simulink model "TPS_Failure_Sys"  (R2020a)
settings: Solver=FixedStepDiscrete  StartTime=0.0  StopTime=10.0  FixedStep=.2  RelTol=1e-3
settings Model: Creator=Administrator  LastModifiedBy=Administrator
settings OptimizationCC: DefaultParameterBehavior=Inlined  EnhancedBackFolding=on  PassReuseOutputArgsAs=Individual arguments  ZeroExternalMemoryAtStartup=off  ZeroInternalMemoryAtStartup=off  OptimizeBlockOrder=speed  DifferentSizesBufferReuse=on  OptimizationCustomize=off  EfficientTunableParamExpr=on
settings DebuggingCC: ParameterTunabilityLossMsg=error
settings HardwareCC: ProdBitPerPointer=32  ProdBitPerSizeT=32  ProdBitPerPtrDiffT=32  ProdLargestAtomicInteger=Long  ProdLargestAtomicFloat=Double  ProdWordSize=32  ProdHWDeviceType=ARM Compatible->ARM Cortex
settings SFSimCC: MATLABDynamicMemAlloc=off
settings RTWCC: SystemTargetFile=ert.tlc  GenCodeOnly=on  TemplateMakefile=ert_default_tmf
settings CodeAppCC: ForceParamTrailComments=on  IgnoreCustomStorageClasses=off  OperatorAnnotations=on  SimulinkDataObjDesc=on  SFDataObjDesc=on  InsertBlockDesc=on
settings ERTTargetCC: TargetLangStandard=C99 (ISO)  GenerateSampleERTMain=on  InlinedParameterPlacement=NonHierarchical  ERTCustomFileTemplate=example_file_process.tlc

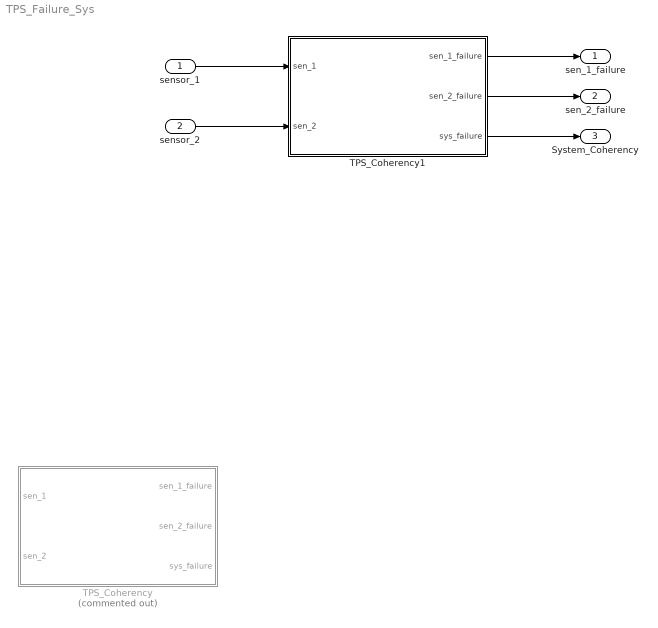
== system TPS_Failure_Sys ==
  sensor_1 : Inport
  sensor_2 : Inport  Port=2
  TPS_Coherency : Stateflow chart  Commented=on  TreatAsAtomicUnit=on
  TPS_Coherency1 : Stateflow chart  TreatAsAtomicUnit=on
  sen_1_failure : Outport
  sen_2_failure : Outport  Port=2
  System_Coherency : Outport  Port=3
  wires:
  sensor_2/1 -> TPS_Coherency1/2(sen_2)
  sensor_1/1 -> TPS_Coherency1/1(sen_1)
  TPS_Coherency1/2(sen_2_failure) -> sen_2_failure/1
  TPS_Coherency1/3(sys_failure) -> System_Coherency/1
  TPS_Coherency1/1(sen_1_failure) -> sen_1_failure/1

== stateflow chart TPS_Failure_Sys/TPS_Coherency1 ==
  state sen2 [parallel]
    settings: executionOrder=3
    (default) -> (junction 112)
    (junction 112) -> (junction 111) [order 1] : [sen_2<.5 || sen_2>4.5]
    sen2 -> (junction 112)
    (junction 111) -> (junction 102) : {sen_2_failure=1}
    (junction 112) -> (junction 105) [order 2] : {sen_2_failure=0}
    (junction 105) -> (junction 102)
    (junction 102) -> (junction 110)
  state sen1 [parallel]
    settings: executionOrder=1
    (default) -> (junction 12)
    (junction 12) -> (junction 14) [order 1] : [sen_1<.5 || sen_1>4.5]
    sen1 -> (junction 12)
    (junction 14) -> (junction 18) : {sen_1_failure=1}
    (junction 12) -> (junction 20) [order 2] : {sen_1_failure=0}
    (junction 20) -> (junction 18)
    (junction 18) -> (junction 23)
  state sys [parallel]
    settings: executionOrder=2
    (default) -> (junction 47)
    (junction 47) -> (junction 51) [order 1] : [sen_1+ sen_2 !=5]
    sys -> (junction 47)
    (junction 51) -> (junction 46) : {sys_failure=1}
    (junction 47) -> (junction 52) [order 2] : {sys_failure=0}
    (junction 52) -> (junction 46)
    (junction 46) -> (junction 55)
  data: sen_1 input double; sen_1_failure output boolean; sen_2_failure output boolean; sen_2 input double; sys_failure output double

== stateflow chart TPS_Failure_Sys/TPS_Coherency ==
  state Failure_Dig
    (default) -> (junction 12)
    (junction 12) -> (junction 14) [order 1] : [sen_1<.5 || sen_1>4.5]
    Failure_Dig -> (junction 12)
    (junction 14) -> (junction 18) : {sen_1_failure=1}
    (junction 12) -> (junction 20) [order 2] : {sen_1_failure=0}
    (junction 20) -> (junction 18)
    (junction 18) -> (junction 23)
    (junction 23) -> (junction 35)
    (junction 35) -> (junction 39) [order 1] : [sen_2<.5 || sen_2>4.5]
    (junction 39) -> (junction 34) : {sen_2_failure =1}
    (junction 35) -> (junction 40) [order 2] : {sen_2_failure=0}
    (junction 40) -> (junction 34)
    (junction 34) -> (junction 43)
    (junction 43) -> (junction 47)
    (junction 47) -> (junction 51) [order 1] : [sen_1+ sen_2 !=5]
    (junction 47) -> (junction 52) [order 2] : {sys_failure=0}
    (junction 51) -> (junction 46) : {sys_failure=1}
    (junction 52) -> (junction 46)
    (junction 46) -> (junction 55)
  data: sen_1 input double; sen_1_failure output boolean; sen_2_failure output boolean; sen_2 input double; sys_failure output double
